simulink model "stateflow_internalfunction"  (R2015b)
settings: Solver=VariableStepAuto  StartTime=0.0  StopTime=10.0  RelTol=1e-3
settings Model: Creator=amyyang  LastModifiedBy=amyyang

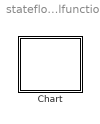
== system stateflow_internalfunction ==
  Chart : Stateflow chart  TreatAsAtomicUnit=on

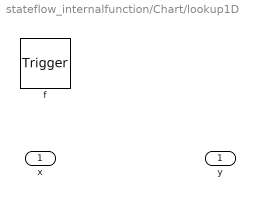
== system stateflow_internalfunction/Chart/lookup1D ==
  x : Inport
  f : TriggerPort  TriggerType=function-call
      settings: CopyFcn=Stateflow.SLINSF.SimulinkMan.removeBlockPreDeleteFcn  PreDeleteFcn=Stateflow.SLINSF.SimulinkMan.unsafePredeleteFcn
  y : Outport

== stateflow chart stateflow_internalfunction/Chart ==
  state y = lookup1D(x) [function]
  note: Incorrect
  state ?
  note: Correct
  state s2
    s2 -> (junction 81) [order 1] : {
        |  a = in * Param;
        |  out = lookup1D(a);
        | }
  (default) -> (junction 91) : {
      |  a = in * Param;
      |  out = lookup1D(a);
      | }
  ? -> s2
  s2 -> ? [order 1]
  data: x function_input; y function_output
